simulink model "testCapteur"  (R2020a)
settings: Solver=VariableStepAuto  StartTime=0.0  StopTime=0.0001  RelTol=1e-3
libraries: fl_lib x7, nesl_utility x3
settings Model: Creator=lucas  LastModifiedBy=Loïc Bouffard

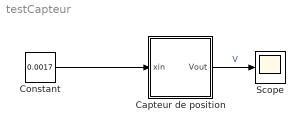
== system testCapteur ==
  Capteur de position : Subsystem  mask{aO=1.2, dE=0.005, gA1=0, Vd1=-1, fc=7234, gA2=0, Vd2=1.1, eL=0.0016, R1=1000, R2=1000, R3=1000, R4=2000}
      mask prompts: aO "Amplitude de l'onde carré de l'oscillateur"; dE "Distance entre les électrodes"; gA1 "Gain du 1er ampli"; Vd1 "Tension décalage 1er ampli"; fc "Fréquence de coupure du filtre"; gA2 "Gain du 2e ampli"; Vd2 "Tension décalage 2e ampli"; eL "Épaisseur de la lame"; R1 "Résistance 1"; R2 "Résistance 2"; R3 "Résistance 3"; R4 "Résistance 4"
  Constant : Constant  Value=0.0017
  Scope : Scope
  wires:
  Capteur de position/1(Vout) -> Scope/1  "V"
  Constant/1 -> Capteur de position/1(xin)

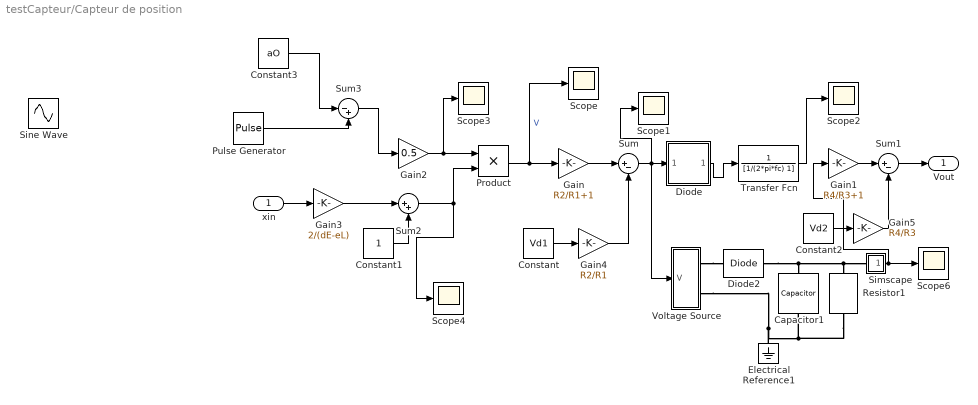
== system testCapteur/Capteur de position ==
  xin : Inport
  Capacitor1 : fl_lib/Electrical/Electrical Elements/Capacitor  c=1 nF  r=1e-6 Ohm  g=0 1/Ohm  i_specify=off  i_priority=None  i=0 A  i_nominal_specify=off  i_nominal_unit=A  i_nominal_value=1  v_specify=off  v_priority=None  v=0 V  v_nominal_specify=off  v_nominal_unit=V  v_nominal_value=1  vc_specify=off  vc_priority=High  vc=0 V  vc_nominal_specify=off  vc_nominal_unit=V  vc_nominal_value=1
  Constant : Constant  Value=Vd1
  Constant1 : Constant
  Constant2 : Constant  Value=Vd2
  Constant3 : Constant  Value=aO
  Diode : Subsystem
  Diode2 : fl_lib/Electrical/Electrical Elements/Diode  Vf=0.6 V  Ron=0.3 Ohm  Goff=1e-8 1/Ohm  i_specify=off  i_priority=None  i=0 A  i_nominal_specify=off  i_nominal_unit=A  i_nominal_value=1  v_specify=off  v_priority=None  v=0 V  v_nominal_specify=off  v_nominal_unit=V  v_nominal_value=1
  Electrical Reference1 : fl_lib/Electrical/Electrical Elements/Electrical Reference
  Gain : Gain  Gain=R2/R1+1
  Gain1 : Gain  Gain=R4/R3+1
  Gain2 : Gain  Gain=0.5
  Gain3 : Gain  Gain=2/(dE-eL)
  Gain4 : Gain  Gain=R2/R1
  Gain5 : Gain  Gain=R4/R3
  Product : Product
  Pulse Generator : DiscretePulseGenerator  PulseType=Time based  Amplitude=2*aO  Period=0.000001  PulseWidth=50
  Resistor1 : fl_lib/Electrical/Electrical Elements/Resistor  R=22 kOhm  i_specify=off  i_priority=None  i=0 A  i_nominal_specify=off  i_nominal_unit=A  i_nominal_value=1  v_specify=off  v_priority=None  v=0 V  v_nominal_specify=off  v_nominal_unit=V  v_nominal_value=1
  Scope{,1..4,6} (6 alike) : Scope
  Simscape : Subsystem
      mask Display: disp('V')
  Sine Wave : Sin  Amplitude=aO  Frequency=2*pi*1000000  SampleTime=0
  Sum : Sum  Inputs=|+-
  Sum1 : Sum  Inputs=|+-
  Sum2 : Sum  Inputs=|++
  Sum3 : Sum  Inputs=|-+
  Transfer Fcn : TransferFcn  Denominator=[1/(2*pi*fc) 1]
  Voltage Source : Subsystem
  Vout : Outport
  wires:
  Gain2/1 -> Scope3/1, Product/1
  Constant1/1 -> Sum2/2
  xin/1 -> Gain3/1
  Gain3/1 -> Sum2/1
  Product/1 -> Scope/1, Gain/1  "V"
  Gain/1 -> Sum/1
  Gain1/1 -> Sum1/1
  Sum/1 -> Scope1/1, Diode/1(In1), Voltage Source/1(V)
  Diode/1(Out1) -> Transfer Fcn/1
  Sum1/1 -> Vout/1
  Constant/1 -> Gain4/1
  Gain4/1 -> Sum/2
  Constant2/1 -> Gain5/1
  Gain5/1 -> Sum1/2
  Sum2/1 -> Product/2, Scope4/1
  Simscape/1(Out) -> Gain1/1, Scope6/1
  Transfer Fcn/1 -> Scope2/1
  Constant3/1 -> Sum3/1
  Pulse Generator/1 -> Sum3/2
  Sum3/1 -> Gain2/1
  connections:
  Voltage Source/RConn1 -- Diode2/LConn1
  Diode2/RConn1 -- Capacitor1/LConn1 -- Simscape/LConn1 -- Resistor1/LConn1
  Voltage Source/RConn2 -- Resistor1/RConn1 -- Capacitor1/RConn1 -- Electrical Reference1/LConn1

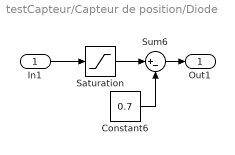
== system testCapteur/Capteur de position/Diode ==
  In1 : Inport
  Constant6 : Constant  Value=0.7
  Saturation : Saturate  UpperLimit=inf  LowerLimit=0.7
  Sum6 : Sum  Inputs=|+-
  Out1 : Outport
  wires:
  Saturation/1 -> Sum6/1
  Constant6/1 -> Sum6/2
  Sum6/1 -> Out1/1
  In1/1 -> Saturation/1

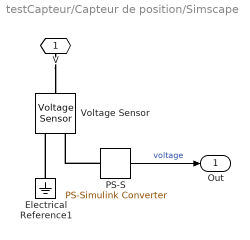
== system testCapteur/Capteur de position/Simscape ==
  Electrical Reference1 : fl_lib/Electrical/Electrical Elements/Electrical Reference
  PS-S : nesl_utility/PS-Simulink Converter  PhysicalDomain=network_engine_domain  SubClassName=ps_output  LeftPortType=input  RightPortType=output  PseudoPeriodic=off  Frequencies=[]  Unit=V  AffineConversion=off
  Voltage Sensor : fl_lib/Electrical/Electrical Sensors/Voltage Sensor
  V : PMIOPort  Side=Left
  Out : Outport  VectorParamsAs1DForOutWhenUnconnected=off
  wires:
  PS-S/1 -> Out/1  "voltage"
  connections:
  PS-S/LConn1 -- Voltage Sensor/RConn1
  V/RConn1 -- Voltage Sensor/LConn1
  Electrical Reference1/LConn1 -- Voltage Sensor/RConn2

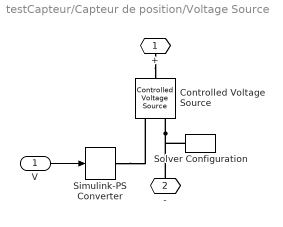
== system testCapteur/Capteur de position/Voltage Source ==
  V : Inport
  Controlled Voltage Source : fl_lib/Electrical/Electrical Sources/Controlled Voltage Source
  Simulink-PS Converter : nesl_utility/Simulink-PS Converter  PhysicalDomain=network_engine_domain  SubClassName=ps_input  LeftPortType=input  RightPortType=output  PseudoPeriodic=off  Frequencies=[]  NoiseDistribution=none  NoiseParameters=[]  Unit=1  AffineConversion=off  FilteringAndDerivatives=zero  SimscapeFilterOrder=1  InputFilterTimeConstant=.001  UdotUserProvided=0
  Solver Configuration : nesl_utility/Solver Configuration  PhysicalDomain=network_engine_domain  SubClassName=solver  LeftPortType=input  RightPortType=generic  Tones=[]  Harmonics=[]  SimulateNoise=off  Profile=off  UseLocalSampling=off  EnableSwitchedLinearOptims=on  FrequencyDomain=off  UseCCode=off  RelTol=0.001  AbsTol=1e-06  MinStep=1e-09  ToWorkspace=off  RevertToSquareIcSolve=off  NumHomotopyIterations=100  PhasorMode=off  PhasorModeNumHarmonics=1  DoDC=off  ResidualTolerance=1e-9  UseLocalSolver=off  LocalSolverChoice=NE_BACKWARD_EULER_ADVANCER  LocalSolverSampleTime=.001  DoFixedCost=off  MaxNonlinIter=3  MaxModeIter=2  LinearAlgebra=auto  EquationFormulation=NE_TIME_EF  DelaysMemoryBudget=1024  AutomaticFiltering=on  FilteringTimeConstant=0.001  PartitionStorageMethod=AS_NEEDED  PartitionMemoryBudget=1024  PartitionMethod=FAST
  + : PMIOPort  Side=Right
  - : PMIOPort  Port=2  Side=Right
  wires:
  V/1 -> Simulink-PS Converter/1
  connections:
  Simulink-PS Converter/RConn1 -- Controlled Voltage Source/RConn1
  Controlled Voltage Source/RConn2 -- -/RConn1 -- Solver Configuration/RConn1
  +/RConn1 -- Controlled Voltage Source/LConn1
